simulink model "dcmotor"  (R2019b)
settings: Solver=VariableStepAuto  StartTime=0.0  StopTime=10  RelTol=1e-4
undefined symbols (not defined in the file or in its folder): fsw, ia_max, ia_min, Jm, k, Ki_i, Ki_n, Kp_i, Kp_n, sigbuilder_block, Ts, Tsc
libraries: fl_lib x16, nesl_utility x9, ee_lib x3, eeDcCurrentController x1, eeDiscretePi x1, eePwmGenerator x1
settings Model: Creator=123  LastModifiedBy=123

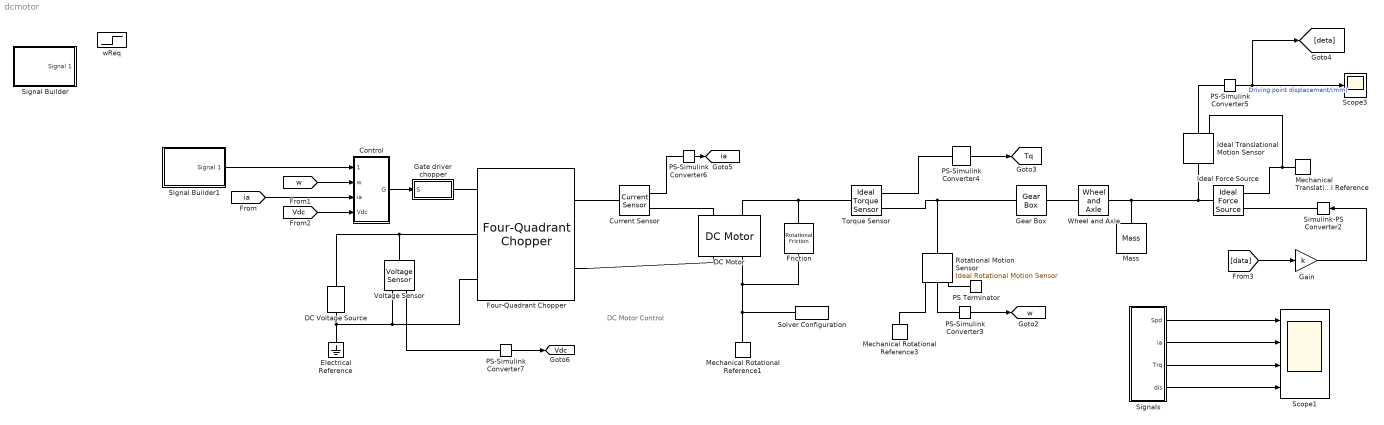
== system dcmotor ==
  note: DC Motor Control
  Control : Subsystem
  Current Sensor : fl_lib/Electrical/Electrical Sensors/Current Sensor
  DC Motor : ee_lib/Electromechanical/Brushed Motors/DC Motor  parameterization=1  Ra=Ra Ohm  La=La H  emf_or_torque=1  Kv=Kb V/(rad/s)  Ki=6.876e-4 N*m/A  T_stall=0.24e-3 N*m  w_max=19100 rpm  w_rated=15000 rpm  P_rated=0.08 W  V_rated=1.5 V  J=Jm kg*m^2  lam_param=1  lam=0 N*m/(rad/s)  i_noload=0 A  V_i_noload=1.5 V  speed0=0 rpm  alpha=3.93e-3 1/K  Tmeas=25 degC  thermal_mass=100 J/K  initial_temperature=25 degC
      settings: SourceProductName=Simscape Electrical
  DC Voltage Source : fl_lib/Electrical/Electrical Sources/DC Voltage Source  v0=15 V
  Electrical Reference : fl_lib/Electrical/Electrical Elements/Electrical Reference
  Four-Quadrant Chopper : ee_lib/Semiconductors & Converters/Converters/Four-Quadrant Chopper  device_type=3  Vf=0.8 V  Ron=0.001 Ohm  Rds=0.001 Ohm  Goff=1e-5 1/Ohm  Vth=0.5 V  Vgt=1 V  Vgt_off=-1 V  Ih=1 A  diode_param=2  diode_Vf=0.8 V  diode_Ron=0.001 Ohm  diode_Goff=1e-5 1/Ohm  diode_C=50 nF  diode_iRM=-235 A  diode_iF=300 A  diode_idot=-50 A/us  diode_trr_param=1  diode_trr_factor=3  diode_trr=15 us  diode_Qrr=1500 s*uA  snubber_type=0  Rs=0.1 Ohm  Cs=1e-7 F
      settings: SourceProductName=Simscape Electrical  SourceProductBaseCode=PS  InternalSimscapePortConfiguration="{\"Bottom\":[],\"Left\":[{\"id\":\"G\",\"label\":\"G\",\"type\":\"foundation.electrical.eight_phase\"},{\"id\":\"p1\",\"label\":\"1+\",\"type\":\"foundation.electrical.electrical\"},{\"id\":\"n1\",\"label\":\"1-\",\"type\":\"foundation.electrical.electrical\"}],\"Right\":[{\"id\":\"p2\",\"label\":\"2+\",\"type\":\"foundation.electrical.electrical\"},{\"id\":\"n2\",\"label\":\"2-\",\"type\":\"foundation.electrical.electrical\"}],\"Top\":[]}"
  Friction : fl_lib/Mechanical/Rotational Elements/Rotational Friction  brkwy_trq=0.02e-3 N*m  brkwy_vel=0.1 rad/s  Col_trq=0.02e-3 N*m  visc_coef=Bm N*m/(rad/s)  w_specify=off  w_priority=None  w=0 rad/s  w_nominal_specify=off  w_nominal_unit=rad/s  w_nominal_value=1  t_specify=off  t_priority=None  t=0 N*m  t_nominal_specify=off  t_nominal_unit=N*m  t_nominal_value=1
      settings: SourceProductName=Simscape
  Gain : Gain  Gain=k
  Gate driver chopper : Subsystem
  Gear Box : fl_lib/Mechanical/Mechanisms/Gear Box  ratio=20  t_in_specify=off  t_in_priority=None  t_in=0 N*m  t_in_nominal_specify=off  t_in_nominal_unit=N*m  t_in_nominal_value=1  t_out_specify=off  t_out_priority=None  t_out=0 N*m  t_out_nominal_specify=off  t_out_nominal_unit=N*m  t_out_nominal_value=1
  Ideal Force Source : fl_lib/Mechanical/Mechanical Sources/Ideal Force Source
  Ideal Translational Motion Sensor : fl_lib/Mechanical/Mechanical Sensors/Ideal Translational Motion Sensor  offset=0 m
  Mass : fl_lib/Mechanical/Translational Elements/Mass  mass=0.1 kg  v_specify=off  v_priority=High  v=0 m/s  v_nominal_specify=off  v_nominal_unit=m/s  v_nominal_value=1  f_specify=off  f_priority=None  f=0 N  f_nominal_specify=off  f_nominal_unit=N  f_nominal_value=1
  Mechanical Rotational Reference1 : fl_lib/Mechanical/Rotational Elements/Mechanical Rotational Reference
  Mechanical Rotational Reference3 : fl_lib/Mechanical/Rotational Elements/Mechanical Rotational Reference
  Mechanical Translational Reference : fl_lib/Mechanical/Translational Elements/Mechanical Translational Reference
  PS Terminator : fl_lib/Physical Signals/Sinks/PS Terminator
      settings: SourceProductName=Simscape
  PS-Simulink Converter3 : nesl_utility/PS-Simulink Converter  PhysicalDomain=network_engine_domain  SubClassName=ps_output  LeftPortType=input  RightPortType=output  PseudoPeriodic=off  Frequencies=[]  Unit=rpm  AffineConversion=off
  PS-Simulink Converter4 : nesl_utility/PS-Simulink Converter  PhysicalDomain=network_engine_domain  SubClassName=ps_output  LeftPortType=input  RightPortType=output  PseudoPeriodic=off  Frequencies=[]  Unit=N*m  AffineConversion=off
  PS-Simulink Converter5 : nesl_utility/PS-Simulink Converter  PhysicalDomain=network_engine_domain  SubClassName=ps_output  LeftPortType=input  RightPortType=output  PseudoPeriodic=off  Frequencies=[]  Unit=inherit  AffineConversion=off
  PS-Simulink Converter6 : nesl_utility/PS-Simulink Converter  PhysicalDomain=network_engine_domain  SubClassName=ps_output  LeftPortType=input  RightPortType=output  PseudoPeriodic=off  Frequencies=[]  Unit=1  AffineConversion=off
  PS-Simulink Converter7 : nesl_utility/PS-Simulink Converter  PhysicalDomain=network_engine_domain  SubClassName=ps_output  LeftPortType=input  RightPortType=output  PseudoPeriodic=off  Frequencies=[]  Unit=V  AffineConversion=off
  Rotational Motion Sensor : fl_lib/Mechanical/Mechanical Sensors/Ideal Rotational Motion Sensor  offset=0 rad
  Scope1 : Scope  NumInputPorts=4
  Scope3 : Scope
  Signal Builder : Subsystem  Tag=STV Subsys  LoadFcn=sigbuilder_block('load');  StartFcn=sigbuilder_block('start');  StopFcn=sigbuilder_block('stop');  ClipboardFcn=sigbuilder_block('clipboard');  mask(Sigbuilder block){tuvar=[0:10]}
      mask help: Simulink:masks:SigbuilderBlock_MD
      mask init:
      | if ~strcmp(get_param(bdroot(gcbh),'SimulationStatus'),'stopped') tuvar = sigbuilder_block('maskInit'); end
      settings: CopyFcn=sigbuilder_block('copy');  DeleteFcn=sigbuilder_block('delete');  ModelCloseFcn=sigbuilder_block('modelClose');  PreSaveFcn=sigbuilder_block('preSave');  PauseFcn=sigbuilder_block('pause');  ContinueFcn=sigbuilder_block('continue');  NameChangeFcn=sigbuilder_block('namechange');  OpenFcn=sigbuilder_block('open',[396 118.2 550.8 400.2 ]);  CloseFcn=sigbuilder_block('close');
      mask Display: plot(0, 0, 100, 100,[2, 2, 32, 32, 2], [68, 8, 8, 68, 68],[32, 2], [38, 38], [32, 19, 2],[53, 60, 44], [32, 17, 17, 2],[16, 16, 31, 31]);txt = getActiveGroup(gcbh);text(2, 100, txt,'verticalAlignment', 'top');
  Signal Builder1 : Subsystem  Tag=STV Subsys  LoadFcn=sigbuilder_block('load');  StartFcn=sigbuilder_block('start');  StopFcn=sigbuilder_block('stop');  ClipboardFcn=sigbuilder_block('clipboard');  mask(Sigbuilder block){tuvar=[0:10]}
      mask help: Simulink:masks:SigbuilderBlock_MD
      mask init:
      | if ~strcmp(get_param(bdroot(gcbh),'SimulationStatus'),'stopped') tuvar = sigbuilder_block('maskInit'); end
      settings: CopyFcn=sigbuilder_block('copy');  DeleteFcn=sigbuilder_block('delete');  ModelCloseFcn=sigbuilder_block('modelClose');  PreSaveFcn=sigbuilder_block('preSave');  PauseFcn=sigbuilder_block('pause');  ContinueFcn=sigbuilder_block('continue');  NameChangeFcn=sigbuilder_block('namechange');  OpenFcn=sigbuilder_block('open',[411.6 178.8 550.8 400.2 ]);  CloseFcn=sigbuilder_block('close');
      mask Display: plot(0, 0, 100, 100,[2, 2, 32, 32, 2], [68, 8, 8, 68, 68],[32, 2], [38, 38], [32, 19, 2],[53, 60, 44], [32, 17, 17, 2],[16, 16, 31, 31]);txt = getActiveGroup(gcbh);text(2, 100, txt,'verticalAlignment', 'top');
  Signals : Subsystem
  Simulink-PS Converter2 : nesl_utility/Simulink-PS Converter  PhysicalDomain=network_engine_domain  SubClassName=ps_input  LeftPortType=input  RightPortType=output  PseudoPeriodic=off  Frequencies=[]  NoiseDistribution=none  NoiseParameters=[]  Unit=1  AffineConversion=off  FilteringAndDerivatives=provide  SimscapeFilterOrder=1  InputFilterTimeConstant=0.001  UdotUserProvided=0
  Solver Configuration : nesl_utility/Solver Configuration  PhysicalDomain=network_engine_domain  SubClassName=solver  LeftPortType=input  RightPortType=generic  Tones=[]  Harmonics=[]  SimulateNoise=off  Profile=off  UseLocalSampling=off  EnableSwitchedLinearOptims=on  FrequencyDomain=off  UseCCode=off  RelTol=0.001  AbsTol=1e-06  MinStep=1e-09  ToWorkspace=off  RevertToSquareIcSolve=off  NumHomotopyIterations=100  PhasorMode=off  PhasorModeNumHarmonics=1  DoDC=off  ResidualTolerance=1e-09  UseLocalSolver=on  LocalSolverChoice=NE_BACKWARD_EULER_ADVANCER  LocalSolverSampleTime=Ts  DoFixedCost=on  MaxNonlinIter=3  MaxModeIter=2  LinearAlgebra=auto  EquationFormulation=NE_TIME_EF  DelaysMemoryBudget=1024  AutomaticFiltering=on  FilteringTimeConstant=0.001  PartitionStorageMethod=AS_NEEDED  PartitionMemoryBudget=1024  PartitionMethod=FAST
  Torque Sensor : fl_lib/Mechanical/Mechanical Sensors/Ideal Torque Sensor
  Voltage Sensor : fl_lib/Electrical/Electrical Sensors/Voltage Sensor
  Wheel and Axle : fl_lib/Mechanical/Mechanisms/Wheel and Axle  R=0.02 m  or=1  t_specify=off  t_priority=None  t=0 N*m  t_nominal_specify=off  t_nominal_unit=N*m  t_nominal_value=1  f_specify=off  f_priority=None  f=0 N  f_nominal_specify=off  f_nominal_unit=N  f_nominal_value=1
      settings: SourceProductName=Simscape
  wReq : Step  Time=2.5  After=1000  SampleTime=0
  tag scope: Tq=global, Vdc=global, ia=global, w=global
  wires:
  [w] -> Control/2(w)
  [ia] -> Control/3(ia)
  [Vdc] -> Control/4(Vdc)
  Signals/2(ia) -> Scope1/2
  Signals/1(Spd) -> Scope1/1
  Signals/3(Trq) -> Scope1/3
  Control/1(G) -> Gate driver chopper/1(S)
  PS-Simulink Converter3/1 -> [w]
  PS-Simulink Converter4/1 -> [Tq]
  PS-Simulink Converter5/1 -> [deta], Scope3/1  "Driving point displacement/(mm)"
  Signals/4(dis) -> Scope1/4
  PS-Simulink Converter6/1 -> [ia]
  PS-Simulink Converter7/1 -> [Vdc]
  [data] -> Gain/1
  Gain/1 -> Simulink-PS Converter2/1
  Signal Builder1/1(Signal 1) -> Control/1(wReq)
  connections:
  Solver Configuration/RConn1 -- DC Motor/RConn2 -- Friction/RConn1 -- Mechanical Rotational Reference1/LConn1
  Four-Quadrant Chopper/LConn2 -- Voltage Sensor/LConn1 -- DC Voltage Source/LConn1
  Friction/LConn1 -- DC Motor/LConn2 -- Torque Sensor/LConn1
  Four-Quadrant Chopper/LConn3 -- Voltage Sensor/RConn2 -- Electrical Reference/LConn1 -- DC Voltage Source/RConn1
  Four-Quadrant Chopper/RConn2 -- DC Motor/RConn1
  Current Sensor/RConn2 -- DC Motor/LConn1
  Gate driver chopper/RConn1 -- Four-Quadrant Chopper/LConn1
  Torque Sensor/RConn1 -- Gear Box/LConn1 -- Rotational Motion Sensor/LConn1
  PS-Simulink Converter3/LConn1 -- Rotational Motion Sensor/RConn2
  Rotational Motion Sensor/RConn1 -- Mechanical Rotational Reference3/LConn1
  Torque Sensor/RConn2 -- PS-Simulink Converter4/LConn1
  PS Terminator/LConn1 -- Rotational Motion Sensor/RConn3
  Ideal Force Source/RConn2 -- Ideal Translational Motion Sensor/RConn1 -- Mechanical Translational Reference/LConn1
  Simulink-PS Converter2/RConn1 -- Ideal Force Source/RConn1
  PS-Simulink Converter5/LConn1 -- Ideal Translational Motion Sensor/RConn2
  Wheel and Axle/LConn1 -- Gear Box/RConn1
  PS-Simulink Converter6/LConn1 -- Current Sensor/RConn1
  Four-Quadrant Chopper/RConn1 -- Current Sensor/LConn1
  PS-Simulink Converter7/LConn1 -- Voltage Sensor/RConn1
  Mass/LConn1 -- Ideal Translational Motion Sensor/LConn1 -- Ideal Force Source/LConn1 -- Wheel and Axle/RConn1

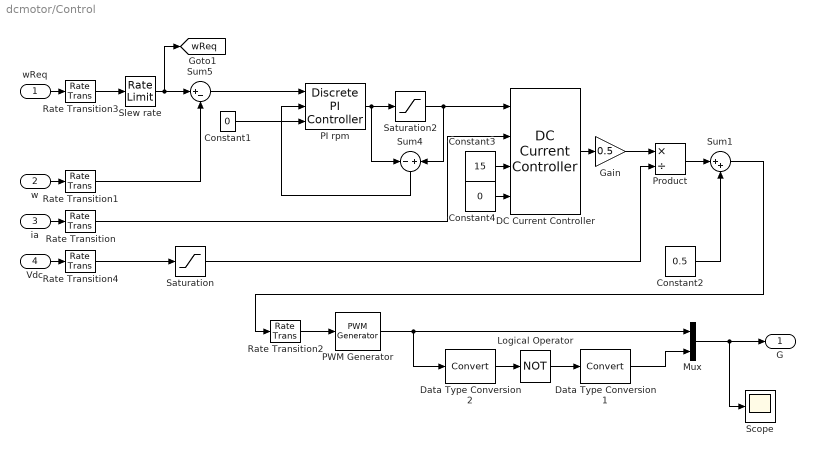
== system dcmotor/Control ==
  wReq : Inport
  w : Inport  Port=2
  ia : Inport  Port=3
  Vdc : Inport  Port=4
  Constant1 : Constant  Value=0  SampleTime=Tsc
  Constant2 : Constant  Value=0.5  SampleTime=Tsc
  Constant3 : Constant  Value=15  SampleTime=Tsc
  Constant4 : Constant  Value=0  SampleTime=Tsc
  DC Current Controller : eeDcCurrentController/DC Current Controller  Kp=Kp_i  Ki=Ki_i  Kaw=Kaw_i  VoltLim=Positive and negative voltage  Ts=Tsc  Tsd=0.001  ActZC=off
      settings: SourceProductName=Simscape Electrical  SourceProductBaseCode=PS
  Data Type Conversion1 : DataTypeConversion
  Data Type Conversion2 : DataTypeConversion
  Gain : Gain  Gain=0.5
  Logical Operator : Logic  Operator=NOT  AllPortsSameDT=off  OutDataTypeStr=boolean
  Mux : Mux  Inputs=2
  PI rpm : eeDiscretePi/Discrete PI Controller  Kp=Kp_n  Ki=Ki_n  Kaw=Kaw_n  x0=0  Ts=Tsc
      settings: SourceProductName=Simscape Electrical  SourceProductBaseCode=PS
  PWM Generator : eePwmGenerator/PWM Generator  CarrCount=Up  Tper=1/fsw  Ts=Ts
      settings: SourceProductName=Simscape Electrical
  Product : Product  Inputs=*/
  Rate Transition{,1,3..4} (4 alike) : RateTransition  OutPortSampleTime=Tsc
  Rate Transition2 : RateTransition  OutPortSampleTime=Ts
  Saturation : Saturate  UpperLimit=20  LowerLimit=0.5
  Saturation2 : Saturate  UpperLimit=ia_max  LowerLimit=ia_min
  Scope : Scope
  Slew rate : RateLimiter  RisingSlewLimit=1000  FallingSlewLimit=-1000  SampleTimeMode=inherited
      settings: AttributesFormatString=2000 rpm/s
  Sum1 : Sum  Inputs=|++
  Sum4 : Sum  Inputs=-+
  Sum5 : Sum  Inputs=|+-
  G : Outport  VectorParamsAs1DForOutWhenUnconnected=off
  tag scope: wReq=global
  wires:
  Constant1/1 -> PI rpm/3
  Sum5/1 -> PI rpm/1
  Saturation/1 -> Product/2
  Sum4/1 -> PI rpm/2
  Saturation2/1 -> DC Current Controller/1, Sum4/2
  wReq/1 -> Rate Transition3/1
  Gain/1 -> Product/1
  Product/1 -> Sum1/1
  w/1 -> Rate Transition1/1
  Slew rate/1 -> Sum5/1, [wReq]
  Vdc/1 -> Rate Transition4/1
  Constant2/1 -> Sum1/2
  Rate Transition3/1 -> Slew rate/1
  ia/1 -> Rate Transition/1
  Rate Transition4/1 -> Saturation/1
  Rate Transition1/1 -> Sum5/2
  DC Current Controller/1 -> Gain/1
  Rate Transition/1 -> DC Current Controller/2
  Constant3/1 -> DC Current Controller/3
  Constant4/1 -> DC Current Controller/4
  PWM Generator/1 -> Mux/1, Data Type Conversion2/1
  Logical Operator/1 -> Data Type Conversion1/1
  Mux/1 -> Scope/1, G/1
  Data Type Conversion2/1 -> Logical Operator/1
  Rate Transition2/1 -> PWM Generator/1
  Data Type Conversion1/1 -> Mux/2
  Sum1/1 -> Rate Transition2/1
  PI rpm/1 -> Sum4/1, Saturation2/1

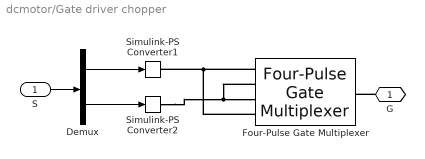
== system dcmotor/Gate driver chopper ==
  S : Inport
  Demux : Demux  Outputs=2
  Four-Pulse Gate Multiplexer : ee_lib/Semiconductors & Converters/Converters/Four-Pulse Gate Multiplexer  R=0 Ohm
      settings: SourceProductName=Simscape Electrical  SourceProductBaseCode=PS  InternalSimscapePortConfiguration="{\"Bottom\":[],\"Left\":[{\"id\":\"G1\",\"label\":\"G1\",\"type\":\"input\"},{\"id\":\"G2\",\"label\":\"G2\",\"type\":\"input\"},{\"id\":\"G3\",\"label\":\"G3\",\"type\":\"input\"},{\"id\":\"G4\",\"label\":\"G4\",\"type\":\"input\"}],\"Right\":[{\"id\":\"p\",\"label\":\"G\",\"type\":\"foundation.electrical.eight_phase\"}],\"Top\":[]}"
  Simulink-PS Converter1 : nesl_utility/Simulink-PS Converter  PhysicalDomain=network_engine_domain  SubClassName=ps_input  LeftPortType=input  RightPortType=output  PseudoPeriodic=off  Frequencies=[]  NoiseDistribution=none  NoiseParameters=[]  Unit=1  AffineConversion=off  FilteringAndDerivatives=zero  SimscapeFilterOrder=1  InputFilterTimeConstant=0.001  UdotUserProvided=1
  Simulink-PS Converter2 : nesl_utility/Simulink-PS Converter  PhysicalDomain=network_engine_domain  SubClassName=ps_input  LeftPortType=input  RightPortType=output  PseudoPeriodic=off  Frequencies=[]  NoiseDistribution=none  NoiseParameters=[]  Unit=1  AffineConversion=off  FilteringAndDerivatives=zero  SimscapeFilterOrder=1  InputFilterTimeConstant=0.001  UdotUserProvided=1
  G : PMIOPort  Side=Right
  wires:
  Demux/2 -> Simulink-PS Converter2/1
  S/1 -> Demux/1
  Demux/1 -> Simulink-PS Converter1/1
  connections:
  Simulink-PS Converter2/RConn1 -- Four-Pulse Gate Multiplexer/LConn2 -- Four-Pulse Gate Multiplexer/LConn3
  Four-Pulse Gate Multiplexer/LConn1 -- Four-Pulse Gate Multiplexer/LConn4 -- Simulink-PS Converter1/RConn1
  G/RConn1 -- Four-Pulse Gate Multiplexer/RConn1

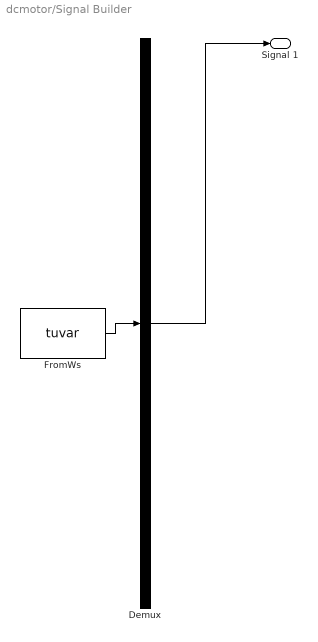
== system dcmotor/Signal Builder ==
  Demux : Demux  Tag=STV Demux  Outputs=1
  FromWs : FromWorkspace  Tag=STV FromWs  VariableName=tuvar  SampleTime=0
      SigBuilderData=|
      | common.afterFinalStr = 'Extrapolate'
      | common.sampleTime = 0
      | dataSet.timeRange = [0 10]
      | dataSet.name = 'Group 1'
      | sbobj.Groups.Name = 'Group 1'
      | sbobj.Groups.Signals.Name = 'Signal 1'
      | sbobj.Groups.Signals.XData = [0 2 2 5 6 6 9 10]
      | sbobj.Groups.Signals.YData = [0 0 1000 1000 1000 0 0 0]
  Signal 1 : Outport  Tag=STV Outport
  wires:
  Demux/1 -> Signal 1/1
  FromWs/1 -> Demux/1

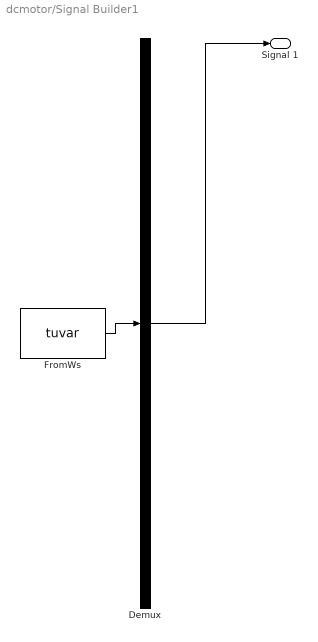
== system dcmotor/Signal Builder1 ==
  Demux : Demux  Tag=STV Demux  Outputs=1
  FromWs : FromWorkspace  Tag=STV FromWs  VariableName=tuvar  SampleTime=0
      SigBuilderData=|
      | common.afterFinalStr = 'Extrapolate'
      | common.sampleTime = 0
      | dataSet.timeRange = [0 10]
      | dataSet.name = 'Group 1'
      | sbobj.Groups.Name = 'Group 1'
      | sbobj.Groups.Signals.Name = 'Signal 1'
      | sbobj.Groups.Signals.XData = [0 2 2 2.5 2.5 6 6 6.5 6.5 10]
      | sbobj.Groups.Signals.YData = [0 10 1000 1000 0 0 -1000 -1000 -10 0]
  Signal 1 : Outport  Tag=STV Outport
  wires:
  Demux/1 -> Signal 1/1
  FromWs/1 -> Demux/1

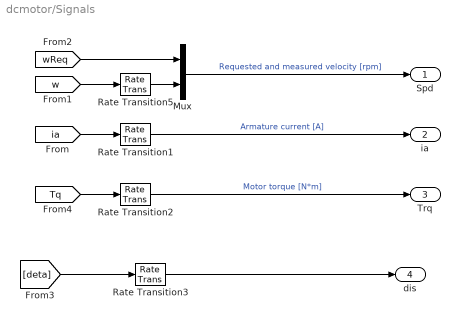
== system dcmotor/Signals ==
  Mux : Mux  Inputs=2
  Rate Transition1 : RateTransition
  Rate Transition2 : RateTransition  OutPortSampleTime=Tsc
  Rate Transition3 : RateTransition  OutPortSampleTime=Tsc
  Rate Transition5 : RateTransition
  Spd : Outport  VectorParamsAs1DForOutWhenUnconnected=off
  ia : Outport  Port=2  VectorParamsAs1DForOutWhenUnconnected=off
  Trq : Outport  Port=3  VectorParamsAs1DForOutWhenUnconnected=off
  dis : Outport  Port=4
  wires:
  Rate Transition2/1 -> Trq/1  "Motor torque [N*m]"
  [ia] -> Rate Transition1/1
  [w] -> Rate Transition5/1
  [Tq] -> Rate Transition2/1
  Rate Transition5/1 -> Mux/2
  Mux/1 -> Spd/1  "Requested and measured velocity [rpm]"
  [wReq] -> Mux/1
  Rate Transition1/1 -> ia/1  "Armature current [A]"
  [deta] -> Rate Transition3/1
  Rate Transition3/1 -> dis/1
